simulink model "Solar PV Pumps Simulation Model"  (R2024b)
settings: Solver=ode4  StartTime=0.0  StopTime=23  RelTol=1e-3
libraries: spsSeriesRLCBranchLib x57, spsIGBTDiodeLib x7, spsAsynchronousMachineSIUnitsLib x6, slpidlib x5, spsCurrentMeasurementLib x3, simulink x2, spsThreePhaseVIMeasurementLib x2, spsabctodq0Lib x2, spsDiodeLib x1, spsVoltageMeasurementLib x1, spsdq0toabcLib x1, spsThreePhaseSourceLib x1
(part 2 of 2)

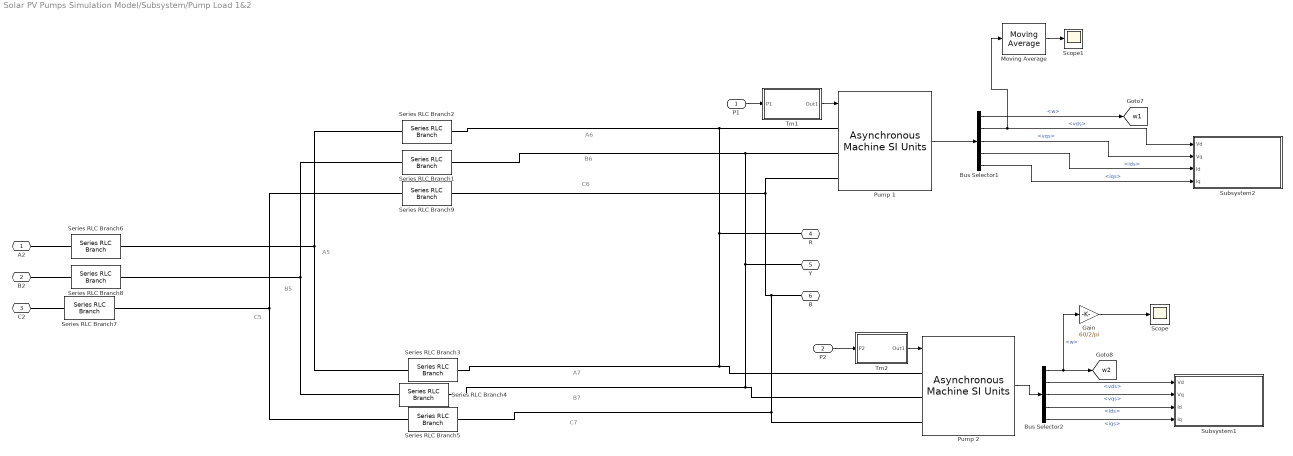
== system Solar PV Pumps Simulation Model/Subsystem/Pump Load 1&2 ==
  note: A5
  note: B5
  note: C5
  note: A6
  note: B6
  note: C6
  note: A7
  note: B7
  note: C7
  P1 : Inport
  P2 : Inport  Port=2
  Bus Selector1 : BusSelector  OutputSignals=w,vds,vqs,ids,iqs
  Bus Selector2 : BusSelector  OutputSignals=w,vds,vqs,ids,iqs
  Gain : Gain  Gain=60/2/pi
  Moving Average : eeGeneralControl/Moving Average  VariantControl=Variant1  LabelModeActiveChoice=Discrete  f=60  x0=0  BufferSize=8192  Ts=-1
      settings: LibrarySourceBlock=ee_sl_lib/General Control/Moving Average
  "Pump 1 " : spsAsynchronousMachineSIUnitsLib/Asynchronous Machine SI Units  RotorType=Squirrel-cage  PresetModel="15:  5.4 HP (4KW)   400 V  50Hz 1430 RPM"  MechanicalLoad=Torque Tm  ShowDetailedParameters=on  ReferenceFrame=Rotor  Units=SI  MeasurementBus=on  NominalParameters=[4000 400 50]  VoltageRatio=1  Stator=[1.405 0.005839]  Rotor=[1.395 0.005839]  Cage1=[0.4155 0.002066]  Cage2=[0.4168 0.0003495]  Lm=0.1722  Mechanical=[0.0131 0.002985 2]  PolePairs=2  InitialConditions=[0 0 0 0 0 0 0 0]  SimulateSaturation=off  Saturation=[14.03593122, 27.81365428, 53.79336849, 72.68890987, 97.98006896, 148.6815601, 215.7428561, 302.9841135, 428.7778367 ; 230, 322, 414, 460, 506, 552, 598, 644, 690]  LoadFlowParameters=1492000  TsPowergui=0  TsBlock=-1  IterativeModel=Trapezoidal non iterative  IterativeDiscreteModel=Trapezoidal non iterative  Pmec=1.492e+006
  Pump 2 : spsAsynchronousMachineSIUnitsLib/Asynchronous Machine SI Units  RotorType=Squirrel-cage  PresetModel="16:  10 HP (7.5KW)  400 V 50Hz 1440 RPM"  MechanicalLoad=Torque Tm  ShowDetailedParameters=on  ReferenceFrame=Rotor  Units=SI  MeasurementBus=on  NominalParameters=[7500 400 50]  VoltageRatio=1  Stator=[0.7384 0.003045]  Rotor=[0.7402 0.003045]  Cage1=[0.4155 0.002066]  Cage2=[0.4168 0.0003495]  Lm=0.1241  Mechanical=[0.0343 0.000503 2]  PolePairs=2  InitialConditions=[0 0 0 0 0 0 0 0]  SimulateSaturation=off  Saturation=[14.03593122, 27.81365428, 53.79336849, 72.68890987, 97.98006896, 148.6815601, 215.7428561, 302.9841135, 428.7778367 ; 230, 322, 414, 460, 506, 552, 598, 644, 690]  LoadFlowParameters=1492000  TsPowergui=0  TsBlock=-1  IterativeModel=Trapezoidal non iterative  IterativeDiscreteModel=Trapezoidal non iterative  Pmec=1.492e+006
  Scope : Scope
  Scope1 : Scope
  Series RLC Branch1 : spsSeriesRLCBranchLib/Series RLC Branch  LConnTagsString=__new0  RConnTagsString=__new0  BranchType=RL  Resistance=0.061540/10  Inductance=1.50E-06  SetiL0=off  InitialCurrent=0  Capacitance=1e-6  Setx0=off  InitialVoltage=0  Measurements=None
  Series RLC Branch2 : spsSeriesRLCBranchLib/Series RLC Branch  LConnTagsString=__new0  RConnTagsString=__new0  BranchType=RL  Resistance=0.061540/10  Inductance=1.50E-06  SetiL0=off  InitialCurrent=0  Capacitance=1e-6  Setx0=off  InitialVoltage=0  Measurements=None
  Series RLC Branch3 : spsSeriesRLCBranchLib/Series RLC Branch  LConnTagsString=__new0  RConnTagsString=__new0  BranchType=RL  Resistance=0.077592/10  Inductance=1.89E-06  SetiL0=off  InitialCurrent=0  Capacitance=1e-6  Setx0=off  InitialVoltage=0  Measurements=None
  Series RLC Branch4 : spsSeriesRLCBranchLib/Series RLC Branch  LConnTagsString=__new0  RConnTagsString=__new0  BranchType=RL  Resistance=0.077592/10  Inductance=1.89E-06  SetiL0=off  InitialCurrent=0  Capacitance=1e-6  Setx0=off  InitialVoltage=0  Measurements=None
  Series RLC Branch5 : spsSeriesRLCBranchLib/Series RLC Branch  LConnTagsString=__new0  RConnTagsString=__new0  BranchType=RL  Resistance=0.077592/10  Inductance=1.89E-06  SetiL0=off  InitialCurrent=0  Capacitance=1e-6  Setx0=off  InitialVoltage=0  Measurements=None
  Series RLC Branch6 : spsSeriesRLCBranchLib/Series RLC Branch  LConnTagsString=__new0  RConnTagsString=__new0  BranchType=RL  Resistance=0.067906/10  Inductance=1.65E-06  SetiL0=off  InitialCurrent=0  Capacitance=1e-6  Setx0=off  InitialVoltage=0  Measurements=None
  Series RLC Branch7 : spsSeriesRLCBranchLib/Series RLC Branch  LConnTagsString=__new0  RConnTagsString=__new0  BranchType=RL  Resistance=0.067906/10  Inductance=1.65E-06  SetiL0=off  InitialCurrent=0  Capacitance=1e-6  Setx0=off  InitialVoltage=0  Measurements=None
  Series RLC Branch8 : spsSeriesRLCBranchLib/Series RLC Branch  LConnTagsString=__new0  RConnTagsString=__new0  BranchType=RL  Resistance=0.067906/10  Inductance=1.65E-06  SetiL0=off  InitialCurrent=0  Capacitance=1e-6  Setx0=off  InitialVoltage=0  Measurements=None
  Series RLC Branch9 : spsSeriesRLCBranchLib/Series RLC Branch  LConnTagsString=__new0  RConnTagsString=__new0  BranchType=RL  Resistance=0.061540/10  Inductance=1.50E-06  SetiL0=off  InitialCurrent=0  Capacitance=1e-6  Setx0=off  InitialVoltage=0  Measurements=None
  Subsystem1 : Subsystem
  Subsystem2 : Subsystem
  Tm1 : Subsystem
  Tm2 : Subsystem
  A2 : PMIOPort  Side=Left
  B2 : PMIOPort  Port=2  Side=Left
  C2 : PMIOPort  Port=3  Side=Left
  R : PMIOPort  Port=4  Side=Right
  Y : PMIOPort  Port=5  Side=Right
  B : PMIOPort  Port=6  Side=Right
  tag scope: w1=global, w2=global
  wires:
  Bus Selector1/1 -> [w1]  "<w>"
  Bus Selector2/1 -> Gain/1, [w2]  "<w>"
  "Pump 1 "/1 -> Bus Selector1/1
  Pump 2/1 -> Bus Selector2/1
  Tm1/1(Out1) -> "Pump 1 "/1
  Tm2/1(Out1) -> Pump 2/1
  Bus Selector2/2 -> Subsystem1/1(Vd)  "<vds>"
  Bus Selector2/3 -> Subsystem1/2(Vq)  "<vqs>"
  Bus Selector2/4 -> Subsystem1/3(Id)  "<ids>"
  Bus Selector2/5 -> Subsystem1/4(Iq)  "<iqs>"
  Bus Selector1/2 -> Moving Average/1, Subsystem2/1(Vd)  "<vds>"
  Bus Selector1/3 -> Subsystem2/2(Vq)  "<vqs>"
  Bus Selector1/4 -> Subsystem2/3(Id)  "<ids>"
  Bus Selector1/5 -> Subsystem2/4(Iq)  "<iqs>"
  Moving Average/1 -> Scope1/1
  Gain/1 -> Scope/1
  P2/1 -> Tm2/1(P2)
  P1/1 -> Tm1/1(P1)
  connections:
  Series RLC Branch8/RConn1 -- Series RLC Branch4/LConn1 -- Series RLC Branch1/LConn1
  Series RLC Branch7/RConn1 -- Series RLC Branch5/LConn1 -- Series RLC Branch9/LConn1
  Series RLC Branch6/RConn1 -- Series RLC Branch3/LConn1 -- Series RLC Branch2/LConn1
  A2/RConn1 -- Series RLC Branch6/LConn1
  Series RLC Branch7/LConn1 -- C2/RConn1
  Series RLC Branch5/RConn1 -- Pump 2/LConn3 -- B/RConn1 -- "Pump 1 "/LConn3 -- Series RLC Branch9/RConn1
  Series RLC Branch1/RConn1 -- Series RLC Branch4/RConn1 -- Pump 2/LConn2 -- Y/RConn1 -- "Pump 1 "/LConn2
  Series RLC Branch2/RConn1 -- Series RLC Branch3/RConn1 -- Pump 2/LConn1 -- R/RConn1 -- "Pump 1 "/LConn1
  Series RLC Branch8/LConn1 -- B2/RConn1

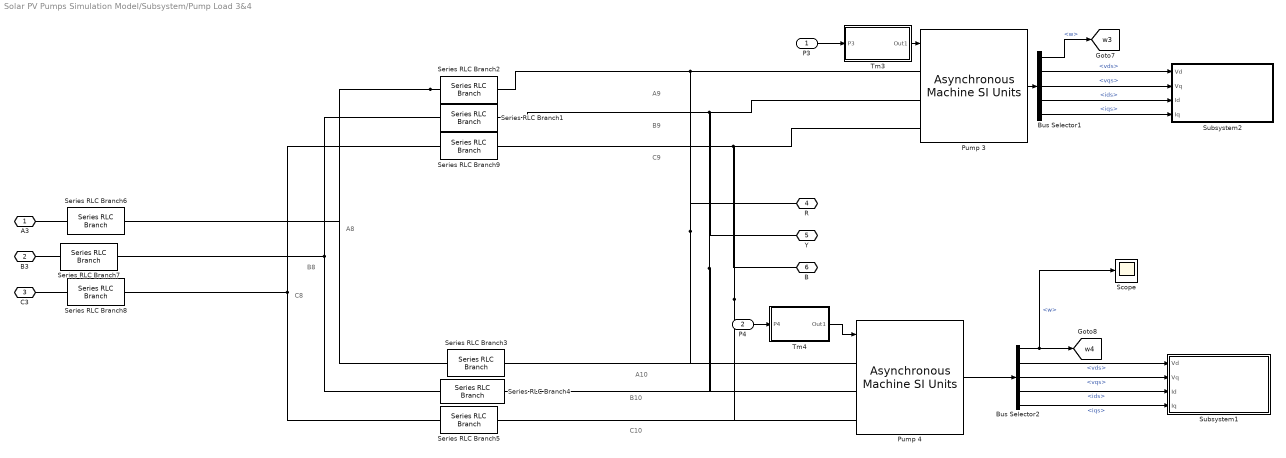
== system Solar PV Pumps Simulation Model/Subsystem/Pump Load 3&4 ==
  note: A8
  note: B8
  note: C8
  note: A9
  note: B9
  note: C9
  note: B10
  note: C10
  note: A10
  P3 : Inport
  P4 : Inport  Port=2
  Bus Selector1 : BusSelector  OutputSignals=w,vds,vqs,ids,iqs
  Bus Selector2 : BusSelector  OutputSignals=w,vds,vqs,ids,iqs
  "Pump 3 " : spsAsynchronousMachineSIUnitsLib/Asynchronous Machine SI Units  RotorType=Squirrel-cage  PresetModel="15:  5.4 HP (4KW)   400 V  50Hz 1430 RPM"  MechanicalLoad=Torque Tm  ShowDetailedParameters=on  ReferenceFrame=Rotor  Units=SI  MeasurementBus=on  NominalParameters=[4000 400 50]  VoltageRatio=1  Stator=[1.405 0.005839]  Rotor=[1.395 0.005839]  Cage1=[0.4155 0.002066]  Cage2=[0.4168 0.0003495]  Lm=0.1722  Mechanical=[0.0131 0.002985 2]  PolePairs=2  InitialConditions=[0 0 0 0 0 0 0 0]  SimulateSaturation=off  Saturation=[14.03593122, 27.81365428, 53.79336849, 72.68890987, 97.98006896, 148.6815601, 215.7428561, 302.9841135, 428.7778367 ; 230, 322, 414, 460, 506, 552, 598, 644, 690]  LoadFlowParameters=1492000  TsPowergui=0  TsBlock=-1  IterativeModel=Trapezoidal non iterative  IterativeDiscreteModel=Trapezoidal non iterative  Pmec=1.492e+006
  Pump 4 : spsAsynchronousMachineSIUnitsLib/Asynchronous Machine SI Units  RotorType=Squirrel-cage  PresetModel="16:  10 HP (7.5KW)  400 V 50Hz 1440 RPM"  MechanicalLoad=Torque Tm  ShowDetailedParameters=on  ReferenceFrame=Rotor  Units=SI  MeasurementBus=on  NominalParameters=[7500 400 50]  VoltageRatio=1  Stator=[0.7384 0.003045]  Rotor=[0.7402 0.003045]  Cage1=[0.4155 0.002066]  Cage2=[0.4168 0.0003495]  Lm=0.1241  Mechanical=[0.0343 0.000503 2]  PolePairs=2  InitialConditions=[0 0 0 0 0 0 0 0]  SimulateSaturation=off  Saturation=[14.03593122, 27.81365428, 53.79336849, 72.68890987, 97.98006896, 148.6815601, 215.7428561, 302.9841135, 428.7778367 ; 230, 322, 414, 460, 506, 552, 598, 644, 690]  LoadFlowParameters=1492000  TsPowergui=0  TsBlock=-1  IterativeModel=Trapezoidal non iterative  IterativeDiscreteModel=Trapezoidal non iterative  Pmec=1.492e+006
  Scope : Scope
  Series RLC Branch1 : spsSeriesRLCBranchLib/Series RLC Branch  LConnTagsString=__new0  RConnTagsString=__new0  BranchType=RL  Resistance=0.070755/10  Inductance=1.72E-06  SetiL0=off  InitialCurrent=0  Capacitance=1e-6  Setx0=off  InitialVoltage=0  Measurements=None
  Series RLC Branch2 : spsSeriesRLCBranchLib/Series RLC Branch  LConnTagsString=__new0  RConnTagsString=__new0  BranchType=RL  Resistance=0.070755/10  Inductance=1.72E-06  SetiL0=off  InitialCurrent=0  Capacitance=1e-6  Setx0=off  InitialVoltage=0  Measurements=None
  Series RLC Branch3 : spsSeriesRLCBranchLib/Series RLC Branch  LConnTagsString=__new0  RConnTagsString=__new0  BranchType=RL  Resistance=0.074107/10  Inductance=1.81E-06  SetiL0=off  InitialCurrent=0  Capacitance=1e-6  Setx0=off  InitialVoltage=0  Measurements=None
  Series RLC Branch4 : spsSeriesRLCBranchLib/Series RLC Branch  LConnTagsString=__new0  RConnTagsString=__new0  BranchType=RL  Resistance=0.074107/10  Inductance=1.81E-06  SetiL0=off  InitialCurrent=0  Capacitance=1e-6  Setx0=off  InitialVoltage=0  Measurements=None
  Series RLC Branch5 : spsSeriesRLCBranchLib/Series RLC Branch  LConnTagsString=__new0  RConnTagsString=__new0  BranchType=RL  Resistance=0.074107/10  Inductance=1.81E-06  SetiL0=off  InitialCurrent=0  Capacitance=1e-6  Setx0=off  InitialVoltage=0  Measurements=None
  Series RLC Branch6 : spsSeriesRLCBranchLib/Series RLC Branch  LConnTagsString=__new0  RConnTagsString=__new0  BranchType=RL  Resistance=0.065855/10  Inductance=1.60E-06  SetiL0=off  InitialCurrent=0  Capacitance=1e-6  Setx0=off  InitialVoltage=0  Measurements=None
  Series RLC Branch7 : spsSeriesRLCBranchLib/Series RLC Branch  LConnTagsString=__new0  RConnTagsString=__new0  BranchType=RL  Resistance=0.065855/10  Inductance=1.60E-06  SetiL0=off  InitialCurrent=0  Capacitance=1e-6  Setx0=off  InitialVoltage=0  Measurements=None
  Series RLC Branch8 : spsSeriesRLCBranchLib/Series RLC Branch  LConnTagsString=__new0  RConnTagsString=__new0  BranchType=RL  Resistance=0.065855/10  Inductance=1.60E-06  SetiL0=off  InitialCurrent=0  Capacitance=1e-6  Setx0=off  InitialVoltage=0  Measurements=None
  Series RLC Branch9 : spsSeriesRLCBranchLib/Series RLC Branch  LConnTagsString=__new0  RConnTagsString=__new0  BranchType=RL  Resistance=0.070755/10  Inductance=1.72E-06  SetiL0=off  InitialCurrent=0  Capacitance=1e-6  Setx0=off  InitialVoltage=0  Measurements=None
  Subsystem1 : Subsystem
  Subsystem2 : Subsystem
  Tm3 : Subsystem
  Tm4 : Subsystem
  A3 : PMIOPort  Side=Left
  B3 : PMIOPort  Port=2  Side=Left
  C3 : PMIOPort  Port=3  Side=Left
  R : PMIOPort  Port=4  Side=Right
  Y : PMIOPort  Port=5  Side=Right
  B : PMIOPort  Port=6  Side=Right
  tag scope: w3=global, w4=global
  wires:
  Bus Selector1/1 -> [w3]  "<w>"
  Bus Selector2/1 -> Scope/1, [w4]  "<w>"
  "Pump 3 "/1 -> Bus Selector1/1
  Pump 4/1 -> Bus Selector2/1
  Tm3/1(Out1) -> "Pump 3 "/1
  Tm4/1(Out1) -> Pump 4/1
  Bus Selector2/2 -> Subsystem1/1(Vd)  "<vds>"
  Bus Selector2/3 -> Subsystem1/2(Vq)  "<vqs>"
  Bus Selector2/4 -> Subsystem1/3(Id)  "<ids>"
  Bus Selector2/5 -> Subsystem1/4(Iq)  "<iqs>"
  Bus Selector1/2 -> Subsystem2/1(Vd)  "<vds>"
  Bus Selector1/3 -> Subsystem2/2(Vq)  "<vqs>"
  Bus Selector1/4 -> Subsystem2/3(Id)  "<ids>"
  Bus Selector1/5 -> Subsystem2/4(Iq)  "<iqs>"
  P3/1 -> Tm3/1(P3)
  P4/1 -> Tm4/1(P4)
  connections:
  Series RLC Branch7/RConn1 -- Series RLC Branch4/LConn1 -- Series RLC Branch1/LConn1
  Series RLC Branch8/RConn1 -- Series RLC Branch5/LConn1 -- Series RLC Branch9/LConn1
  Series RLC Branch2/LConn1 -- Series RLC Branch3/LConn1 -- Series RLC Branch6/RConn1
  Series RLC Branch8/LConn1 -- C3/RConn1
  Series RLC Branch9/RConn1 -- Series RLC Branch5/RConn1 -- Pump 4/LConn3 -- B/RConn1 -- "Pump 3 "/LConn3
  Series RLC Branch1/RConn1 -- Series RLC Branch4/RConn1 -- Pump 4/LConn2 -- Y/RConn1 -- "Pump 3 "/LConn2
  Series RLC Branch2/RConn1 -- Series RLC Branch3/RConn1 -- Pump 4/LConn1 -- R/RConn1 -- "Pump 3 "/LConn1
  Series RLC Branch7/LConn1 -- B3/RConn1
  A3/RConn1 -- Series RLC Branch6/LConn1

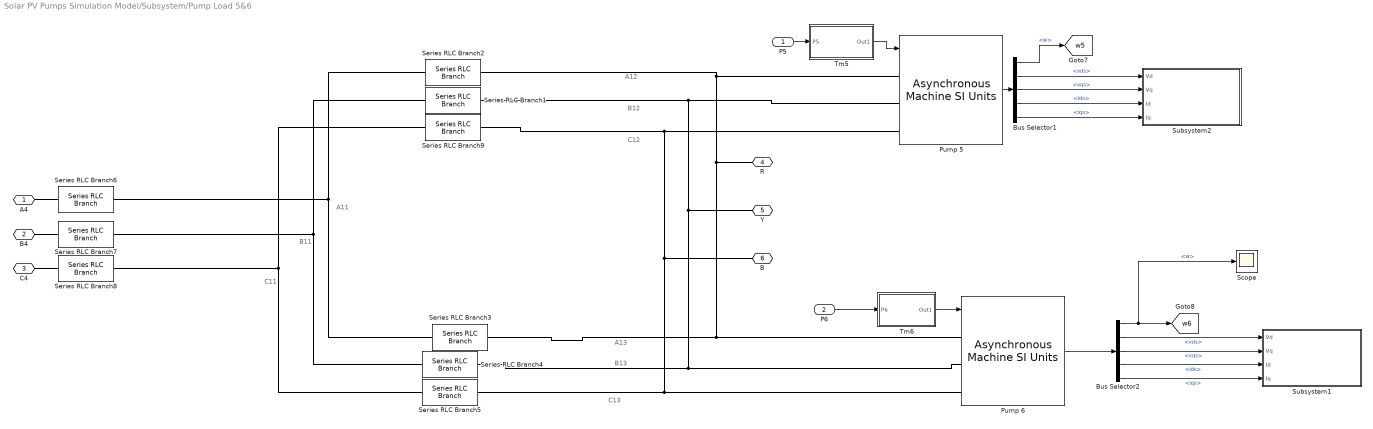
== system Solar PV Pumps Simulation Model/Subsystem/Pump Load 5&6 ==
  note: A11
  note: B11
  note: C11
  note: B12
  note: C12
  note: A12
  note: B13
  note: C13
  note: A13
  P5 : Inport
  P6 : Inport  Port=2
  Bus Selector1 : BusSelector  OutputSignals=w,vds,vqs,ids,iqs
  Bus Selector2 : BusSelector  OutputSignals=w,vds,vqs,ids,iqs
  "Pump 5 " : spsAsynchronousMachineSIUnitsLib/Asynchronous Machine SI Units  RotorType=Squirrel-cage  PresetModel="15:  5.4 HP (4KW)   400 V  50Hz 1430 RPM"  MechanicalLoad=Torque Tm  ShowDetailedParameters=on  ReferenceFrame=Rotor  Units=SI  MeasurementBus=on  NominalParameters=[4000 400 50]  VoltageRatio=1  Stator=[1.405 0.005839]  Rotor=[1.395 0.005839]  Cage1=[0.4155 0.002066]  Cage2=[0.4168 0.0003495]  Lm=0.1722  Mechanical=[0.0131 0.002985 2]  PolePairs=2  InitialConditions=[0 0 0 0 0 0 0 0]  SimulateSaturation=off  Saturation=[14.03593122, 27.81365428, 53.79336849, 72.68890987, 97.98006896, 148.6815601, 215.7428561, 302.9841135, 428.7778367 ; 230, 322, 414, 460, 506, 552, 598, 644, 690]  LoadFlowParameters=1492000  TsPowergui=0  TsBlock=-1  IterativeModel=Trapezoidal non iterative  IterativeDiscreteModel=Trapezoidal non iterative  Pmec=1.492e+006
  Pump 6 : spsAsynchronousMachineSIUnitsLib/Asynchronous Machine SI Units  RotorType=Squirrel-cage  PresetModel="16:  10 HP (7.5KW)  400 V 50Hz 1440 RPM"  MechanicalLoad=Torque Tm  ShowDetailedParameters=on  ReferenceFrame=Rotor  Units=SI  MeasurementBus=on  NominalParameters=[7500 400 50]  VoltageRatio=1  Stator=[0.7384 0.003045]  Rotor=[0.7402 0.003045]  Cage1=[0.4155 0.002066]  Cage2=[0.4168 0.0003495]  Lm=0.1241  Mechanical=[0.0343 0.000503 2]  PolePairs=2  InitialConditions=[0 0 0 0 0 0 0 0]  SimulateSaturation=off  Saturation=[14.03593122, 27.81365428, 53.79336849, 72.68890987, 97.98006896, 148.6815601, 215.7428561, 302.9841135, 428.7778367 ; 230, 322, 414, 460, 506, 552, 598, 644, 690]  LoadFlowParameters=1492000  TsPowergui=0  TsBlock=-1  IterativeModel=Trapezoidal non iterative  IterativeDiscreteModel=Trapezoidal non iterative  Pmec=1.492e+006
  Scope : Scope
  Series RLC Branch{1..5,9} (6 alike) : spsSeriesRLCBranchLib/Series RLC Branch  LConnTagsString=__new0  RConnTagsString=__new0  BranchType=RL  Resistance=0.046421/10  Inductance=1.13E-06  SetiL0=off  InitialCurrent=0  Capacitance=1e-6  Setx0=off  InitialVoltage=0  Measurements=None
  Series RLC Branch6 : spsSeriesRLCBranchLib/Series RLC Branch  LConnTagsString=__new0  RConnTagsString=__new0  BranchType=RL  Resistance=0.094970/10  Inductance=2.31E-06  SetiL0=off  InitialCurrent=0  Capacitance=1e-6  Setx0=off  InitialVoltage=0  Measurements=None
  Series RLC Branch7 : spsSeriesRLCBranchLib/Series RLC Branch  LConnTagsString=__new0  RConnTagsString=__new0  BranchType=RL  Resistance=0.094970/10  Inductance=2.31E-06  SetiL0=off  InitialCurrent=0  Capacitance=1e-6  Setx0=off  InitialVoltage=0  Measurements=None
  Series RLC Branch8 : spsSeriesRLCBranchLib/Series RLC Branch  LConnTagsString=__new0  RConnTagsString=__new0  BranchType=RL  Resistance=0.094970/10  Inductance=2.31E-06  SetiL0=off  InitialCurrent=0  Capacitance=1e-6  Setx0=off  InitialVoltage=0  Measurements=None
  Subsystem1 : Subsystem
  Subsystem2 : Subsystem
  Tm5 : Subsystem
  Tm6 : Subsystem
  A4 : PMIOPort  Side=Left
  B4 : PMIOPort  Port=2  Side=Left
  C4 : PMIOPort  Port=3  Side=Left
  R : PMIOPort  Port=4  Side=Right
  Y : PMIOPort  Port=5  Side=Right
  B : PMIOPort  Port=6  Side=Right
  tag scope: w5=global, w6=global
  wires:
  Bus Selector1/1 -> [w5]  "<w>"
  Bus Selector2/1 -> Scope/1, [w6]  "<w>"
  "Pump 5 "/1 -> Bus Selector1/1
  Pump 6/1 -> Bus Selector2/1
  Tm5/1(Out1) -> "Pump 5 "/1
  Tm6/1(Out1) -> Pump 6/1
  Bus Selector2/2 -> Subsystem1/1(Vd)  "<vds>"
  Bus Selector2/3 -> Subsystem1/2(Vq)  "<vqs>"
  Bus Selector2/4 -> Subsystem1/3(Id)  "<ids>"
  Bus Selector2/5 -> Subsystem1/4(Iq)  "<iqs>"
  Bus Selector1/2 -> Subsystem2/1(Vd)  "<vds>"
  Bus Selector1/3 -> Subsystem2/2(Vq)  "<vqs>"
  Bus Selector1/4 -> Subsystem2/3(Id)  "<ids>"
  Bus Selector1/5 -> Subsystem2/4(Iq)  "<iqs>"
  P6/1 -> Tm6/1(P6)
  P5/1 -> Tm5/1(P5)
  connections:
  Series RLC Branch7/RConn1 -- Series RLC Branch4/LConn1 -- Series RLC Branch1/LConn1
  Series RLC Branch8/RConn1 -- Series RLC Branch5/LConn1 -- Series RLC Branch9/LConn1
  Series RLC Branch2/LConn1 -- Series RLC Branch3/LConn1 -- Series RLC Branch6/RConn1
  A4/RConn1 -- Series RLC Branch6/LConn1
  Series RLC Branch8/LConn1 -- C4/RConn1
  Series RLC Branch9/RConn1 -- Series RLC Branch5/RConn1 -- Pump 6/LConn3 -- B/RConn1 -- "Pump 5 "/LConn3
  Series RLC Branch1/RConn1 -- Y/RConn1 -- Series RLC Branch4/RConn1 -- Pump 6/LConn2 -- "Pump 5 "/LConn2
  Series RLC Branch7/LConn1 -- B4/RConn1
  Series RLC Branch2/RConn1 -- R/RConn1 -- Series RLC Branch3/RConn1 -- Pump 6/LConn1 -- "Pump 5 "/LConn1

== system Solar PV Pumps Simulation Model/Subsystem/Pump Load 1&2/Subsystem1 ==
  Vd : Inport
  Vq : Inport  Port=2
  Id : Inport  Port=3
  Iq : Inport  Port=4
  Add : Sum
  Gain : Gain  Gain=3/2
  Product : Product
  Product1 : Product
  tag scope: P_pump2=global
  wires:
  Iq/1 -> Product1/2
  Product1/1 -> Add/2
  Vq/1 -> Product1/1
  Vd/1 -> Product/1
  Product/1 -> Add/1
  Add/1 -> Gain/1
  Id/1 -> Product/2
  Gain/1 -> [P_pump2]

== system Solar PV Pumps Simulation Model/Subsystem/Pump Load 1&2/Subsystem2 ==
  Vd : Inport
  Vq : Inport  Port=2
  Id : Inport  Port=3
  Iq : Inport  Port=4
  Add : Sum
  Gain : Gain  Gain=3/2
  Product : Product
  Product1 : Product
  Scope : Scope
  tag scope: P_pump1=global
  wires:
  Vq/1 -> Product1/1
  Iq/1 -> Product1/2
  Vd/1 -> Product/1
  Id/1 -> Product/2
  Product/1 -> Add/1
  Product1/1 -> Add/2
  Add/1 -> Gain/1
  Gain/1 -> Scope/1, [P_pump1]

== system Solar PV Pumps Simulation Model/Subsystem/Pump Load 1&2/Tm1 ==
  P1 : Inport
  Constant2 : Constant  Value=0.0011929622
  MATLAB Function : MATLAB Function  TreatAsAtomicUnit=on
  Product : Product
  Square : Math  Operator=square
  Out1 : Outport
  wires:
  Constant2/1 -> Product/2
  Square/1 -> Product/1
  Product/1 -> Out1/1
  MATLAB Function/1(w) -> Square/1
  P1/1 -> MATLAB Function/1(Load)

== system Solar PV Pumps Simulation Model/Subsystem/Pump Load 1&2/Tm2 ==
  P2 : Inport
  Constant3 : Constant  Value=0.002190527
  MATLAB Function : MATLAB Function  TreatAsAtomicUnit=on
  Product1 : Product
  Square1 : Math  Operator=square
  Out1 : Outport
  wires:
  Square1/1 -> Product1/1
  MATLAB Function/1(w) -> Square1/1
  Product1/1 -> Out1/1
  Constant3/1 -> Product1/2
  P2/1 -> MATLAB Function/1(Load)

== system Solar PV Pumps Simulation Model/Subsystem/Pump Load 3&4/Subsystem1 ==
  Vd : Inport
  Vq : Inport  Port=2
  Id : Inport  Port=3
  Iq : Inport  Port=4
  Add : Sum
  Gain : Gain  Gain=3/2
  Product : Product
  Product1 : Product
  tag scope: P_pump4=global
  wires:
  Iq/1 -> Product1/2
  Product1/1 -> Add/2
  Vq/1 -> Product1/1
  Vd/1 -> Product/1
  Product/1 -> Add/1
  Add/1 -> Gain/1
  Id/1 -> Product/2
  Gain/1 -> [P_pump4]

== system Solar PV Pumps Simulation Model/Subsystem/Pump Load 3&4/Subsystem2 ==
  Vd : Inport
  Vq : Inport  Port=2
  Id : Inport  Port=3
  Iq : Inport  Port=4
  Add : Sum
  Gain : Gain  Gain=3/2
  Product : Product
  Product1 : Product
  tag scope: P_pump3=global
  wires:
  Vq/1 -> Product1/1
  Iq/1 -> Product1/2
  Vd/1 -> Product/1
  Id/1 -> Product/2
  Product/1 -> Add/1
  Product1/1 -> Add/2
  Add/1 -> Gain/1
  Gain/1 -> [P_pump3]

== system Solar PV Pumps Simulation Model/Subsystem/Pump Load 3&4/Tm3 ==
  P3 : Inport
  Constant2 : Constant  Value=0.0011929622
  MATLAB Function : MATLAB Function  TreatAsAtomicUnit=on
  Product : Product
  Square : Math  Operator=square
  Out1 : Outport
  wires:
  Constant2/1 -> Product/2
  Square/1 -> Product/1
  Product/1 -> Out1/1
  MATLAB Function/1(w) -> Square/1
  P3/1 -> MATLAB Function/1(Load)

== system Solar PV Pumps Simulation Model/Subsystem/Pump Load 3&4/Tm4 ==
  P4 : Inport
  Constant3 : Constant  Value=0.002190527
  MATLAB Function : MATLAB Function  TreatAsAtomicUnit=on
  Product1 : Product
  Square1 : Math  Operator=square
  Out1 : Outport
  wires:
  Square1/1 -> Product1/1
  Product1/1 -> Out1/1
  Constant3/1 -> Product1/2
  MATLAB Function/1(w) -> Square1/1
  P4/1 -> MATLAB Function/1(Load)

== system Solar PV Pumps Simulation Model/Subsystem/Pump Load 5&6/Subsystem1 ==
  Vd : Inport
  Vq : Inport  Port=2
  Id : Inport  Port=3
  Iq : Inport  Port=4
  Add : Sum
  Gain : Gain  Gain=3/2
  Product : Product
  Product1 : Product
  tag scope: P_pump6=global
  wires:
  Iq/1 -> Product1/2
  Product1/1 -> Add/2
  Vq/1 -> Product1/1
  Vd/1 -> Product/1
  Product/1 -> Add/1
  Add/1 -> Gain/1
  Id/1 -> Product/2
  Gain/1 -> [P_pump6]

== system Solar PV Pumps Simulation Model/Subsystem/Pump Load 5&6/Subsystem2 ==
  Vd : Inport
  Vq : Inport  Port=2
  Id : Inport  Port=3
  Iq : Inport  Port=4
  Add : Sum
  Gain : Gain  Gain=3/2
  Product : Product
  Product1 : Product
  tag scope: P_pump5=global
  wires:
  Vq/1 -> Product1/1
  Iq/1 -> Product1/2
  Vd/1 -> Product/1
  Id/1 -> Product/2
  Product/1 -> Add/1
  Product1/1 -> Add/2
  Add/1 -> Gain/1
  Gain/1 -> [P_pump5]

== system Solar PV Pumps Simulation Model/Subsystem/Pump Load 5&6/Tm5 ==
  P5 : Inport
  Constant2 : Constant  Value=0.0011929622
  MATLAB Function : MATLAB Function  TreatAsAtomicUnit=on
  Product : Product
  Square : Math  Operator=square
  Out1 : Outport
  wires:
  Constant2/1 -> Product/2
  Square/1 -> Product/1
  Product/1 -> Out1/1
  MATLAB Function/1(w) -> Square/1
  P5/1 -> MATLAB Function/1(Load)

== system Solar PV Pumps Simulation Model/Subsystem/Pump Load 5&6/Tm6 ==
  P6 : Inport
  Constant3 : Constant  Value=0.002190527
  MATLAB Function : MATLAB Function  TreatAsAtomicUnit=on
  Product1 : Product
  Square1 : Math  Operator=square
  Out1 : Outport
  wires:
  Square1/1 -> Product1/1
  Product1/1 -> Out1/1
  Constant3/1 -> Product1/2
  MATLAB Function/1(w) -> Square1/1
  P6/1 -> MATLAB Function/1(Load)

== matlab function Solar PV Pumps Simulation Model/Subsystem/Pump Load 1&2/Tm1/MATLAB Function ==
  data: Load input; w output
function w = Speed_Input(Load)

  
    P_rated = 4000
    omega_rated = 1430*2*pi/60
    % 1. Power fraction
    p_frac = Load;

    % 2. Safety clamp (avoid negative / noise issues)
    p_frac = max(0.05, min(1.5, p_frac));

    % 3. Affinity law mapping
    w_frac = p_frac^(1/3);

    % 4. Speed command
    w = omega_rated * w_frac;

end

== matlab function Solar PV Pumps Simulation Model/MPPT/MATLAB Function ==
  data: P input; Vref output; V input
function Vref = fcn(P, V)

% P&O MPPT Algorithm (Improved Version)

% ---- USER PARAMETERS ----
Vref_initial = 750;     % Initial guess near expected MPP (~800 V)
Vrefmax = 900;         % Upper voltage limit
Vrefmin = 500;         % Lower voltage limit
deltaV = 1;            % Step size (can tune: 5–10 for high voltage systems)
epsilon = 1e-3;        % Deadband for power change

% ---- PERSISTENT VARIABLES ----
persistent Vold Pold Vrefold

if isempty(Vold)
    Vold = V;
    Pold = P;
    Vrefold = Vref_initial;
end

% ---- COMPUTE DIFFERENCES ----
dV = V - Vold;
dP = P - Pold;

% ---- P&O LOGIC ----
if abs(dP) < epsilon
    % Very small change → stay at same point
    Vref = Vrefold;

else
    if dP > 0
        if dV >= 0
            Vref = Vrefold + deltaV;
        else
            Vref = Vrefold - deltaV;
        end
    else
        if dV < 0
            Vref = Vrefold + deltaV;
        else
            Vref = Vrefold - deltaV;
        end
    end
end

% ---- SATURATION (IMPORTANT) ----
Vref = min(max(Vref, Vrefmin), Vrefmax);

% ---- UPDATE MEMORY ----
Vrefold = Vref;
Vold = V;
Pold = P;

end

== matlab function Solar PV Pumps Simulation Model/Subsystem/Pump Load 1&2/Tm2/MATLAB Function ==
  data: Load input; w output
function w = Speed_Input(Load)

    
    P_rated = 7500
    omega_rated = 1440*2*pi/60
    % 1. Power fraction
    p_frac = Load;

    % 2. Safety clamp (avoid negative / noise issues)
    p_frac = max(0.05, min(1.5, p_frac));

    % 3. Affinity law mapping
    w_frac = p_frac^(1/3);

    % 4. Speed command
    w = omega_rated * w_frac;

end

== matlab function Solar PV Pumps Simulation Model/Subsystem/Pump Load 5&6/Tm6/MATLAB Function ==
  data: Load input; w output
function w = Speed_Input(Load)

    
    P_rated = 7500
    omega_rated = 1440*2*pi/60
    % 1. Power fraction
    p_frac = Load;

    % 2. Safety clamp (avoid negative / noise issues)
    p_frac = max(0.05, min(1.5, p_frac));

    % 3. Affinity law mapping
    w_frac = p_frac^(1/3);

    % 4. Speed command
    w = omega_rated * w_frac;

end

== matlab function Solar PV Pumps Simulation Model/Subsystem/Pump Load 3&4/Tm4/MATLAB Function ==
  data: Load input; w output
function w = Speed_Input(Load)

    
    P_rated = 7500
    omega_rated = 1440*2*pi/60
    % 1. Power fraction
    p_frac = Load;

    % 2. Safety clamp (avoid negative / noise issues)
    p_frac = max(0.05, min(1.5, p_frac));

    % 3. Affinity law mapping
    w_frac = p_frac^(1/3);

    % 4. Speed command
    w = omega_rated * w_frac;

end

== matlab function Solar PV Pumps Simulation Model/Subsystem/Pump Load 3&4/Tm3/MATLAB Function ==
  data: Load input; w output
function w = Speed_Input(Load)

    
    P_rated = 4000
    omega_rated = 1430*2*pi/60
    % 1. Power fraction
    p_frac = Load;

    % 2. Safety clamp (avoid negative / noise issues)
    p_frac = max(0.05, min(1.5, p_frac));

    % 3. Affinity law mapping
    w_frac = p_frac^(1/3);

    % 4. Speed command
    w = omega_rated * w_frac;

end

== matlab function Solar PV Pumps Simulation Model/Subsystem/Pump Load 5&6/Tm5/MATLAB Function ==
  data: Load input; w output
function w = Speed_Input(Load)

    
    P_rated = 4000
    omega_rated = 1430*2*pi/60
    % 1. Power fraction
    p_frac = Load;

    % 2. Safety clamp (avoid negative / noise issues)
    p_frac = max(0.05, min(1.5, p_frac));

    % 3. Affinity law mapping
    w_frac = p_frac^(1/3);

    % 4. Speed command
    w = omega_rated * w_frac;

end
